simulink model "Steuerung_Modell"  (R2021a)
settings: Solver=FixedStepAuto  StartTime=0.0  StopTime=inf  FixedStep=0.01  MaxStep=0.01  RelTol=1e-3
libraries: simulink x2
settings Model: EnablePacing=on  PacingRate=1.400000  Creator=nymla  LastModifiedBy=nymla

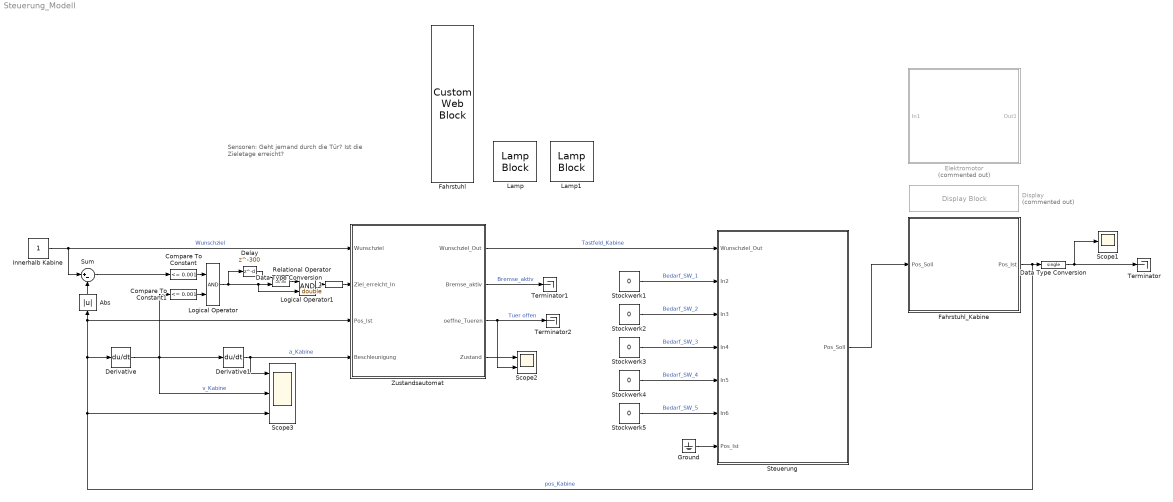
== system Steuerung_Modell ==
  note: Sensoren:
      | Geht jemand durch die Tür?
      | Ist die Zieletage erreicht?
  Abs : Abs
  Compare To Constant : simulink/Logic and Bit Operations/Compare To Constant  relop=<=  const=0.001  OutDataTypeStr=boolean
  Compare To Constant1 : simulink/Logic and Bit Operations/Compare To Constant  relop=<=  const=0.001  OutDataTypeStr=boolean
  Data Type Conversion : DataTypeConversion  OutDataTypeStr=single  RndMeth=Round
  Data Type Conversion1 : DataTypeConversion  OutDataTypeStr=double
  Delay : Delay  DelayLength=300  InitialCondition=1
  Derivative : Derivative
  Derivative1 : Derivative
  Display : DisplayBlock  Commented=on  LabelPosition=Hide  Format=short  Transparency=1
  Elektromotor : Subsystem  Commented=on
  Fahrstuhl : CustomWebBlock  LabelPosition=Hide  ShowInitialText=on  Configuration="{\"components\":[{\"name\":\"LinearScaleComponent\",\"settings\":{\"bounds\":{\"max\":5,\"min\":0,\"tickInterval\":\"auto\"},\"internalTickHeightScaleFactor\":0.5,\"labelColor\":[255,255,200],\"labelFont\":{\"font\":\"Arial\",\"fontSize\":12},\"labelTransparency\":1,\"needleImage\":{\"size\":[21,75],\"src\":\"data:image\\/svg+xml;base64,PHN2ZyB4bWxucz0iaHR0cDovL3d3dy53My5vcmcvMjAwMC9zdmciIHhtbG5zOnhsaW5rPSJodHRwOi8vd3d3LnczLm9yZy8xOTk5L3hsaW5rIiB2aWV3Qm94PSIwIDAgMjEgNzUiPjxkZWZzPjxzdHlsZT4uY2xzLTF7ZmlsbDpub25lO30uY2xzLTJ7aXNvbGF0aW9uOmlzb2xhdGU7fS5jbHMtM3tjbGlwLXBhdGg6dXJsKCNjbGlwLXBhdGgpO30uY2xzLTR7b3BhY2l0eTowLjM7bWl4LWJsZW5kLW1vZGU6bXVsdGlwbHk7fS5jbHMtNXtmaWxsOiNlYjI2Mjk7fTwvc3R5bGU+PGNsaXBQYXRoIGlkPSJjbGlwLXBhdGgiIHRyYW5zZm9y ...(+1928 chars)\",\"srcOrientation\":\"horizontal\"},\"needleOffset\":[-0.01094391244870041,0],\"needleSize\":{\"height\":0.11960078534031414,\"width\":0.7589285714285714},\"position\":[0.015887605042016806,0.06986607142857143,0.8,0.9641544117647058],\"scaleColors\":[],\"scaleColorsSize\":0.2,\"showLabels\":1,\"showMinorTicks\":0,\"showSpanLine\":1,\"showTicks\":1,\"tickColor\":[252,252,197],\"tickTransparency\":1,\"valueBarColor\":[23,89,176],\"valueBarOffset\":0,\"valueBarSize\":0.23,\"valueBarTransparency\":1}},{\"name\":\"BackgroundImageComponent\",\"settings\":{\"image\":{\"size\":[101,380],\"src\":\"data:image\\/svg+xml;base64,PHN2ZyB4bWxucz0iaHR0cDovL3d3dy53My5vcmcvMjAwMC9zdmciIHZpZXdCb3g9IjAgMCAxMDEgMzgwIj48ZGVmcz48c3R5bGU+LmNscy0xe2ZpbGw6IzAwMmI0Mjt9LmNscy0ye2ZpbGw6IzQyNzA4Mjt9LmNscy0ze2ZpbGw6IzdjYTBiMjt9PC9zdHlsZT48L2RlZnM+PHRpdGxlPnZlcnRpY2FsX2dhdWdlX2JhY2tncm91bmRfMTwvdGl0bGU+PGcgaWQ9IkxheWVyXzIiIGRhdGEtbmFtZT0iTGF5ZXIgMiI+PGcgaWQ9IkxheWVyXzEtMiIgZGF0YS1uYW1lPSJMYXllciAxIj48cmVjdCBjbGFzcz0iY2xzLTEiIHg9IjExIiB5PSIxMSIgd2lkdGg9Ijc5IiBoZWlnaHQ9IjM1OCIvPjxwYXRoIGNsYXNzPSJjbHMtMiIgZD0iTTkzLDhIOFYzNzJIOTNaTTExLDM2OVYxMUg5MFYzNjlaIi8+PHBhdGggY2xhc3M9ImNscy0zIiBkPSJNMTAxLDBIMFYzODBIMTAxWk04LDM3MlY4SDkzVjM3MloiLz48L2c+PC9nPjwvc3ZnPg==\",\"srcOrientation\":\"vertical\"},\"position\":[0,0,1,1],\"scaleMode\":\"0\"}},{\"name\":\"ForegroundImageComponent\",\"settings\":{\"image\":{\"size\":[0,0],\"src\":\"default\",\"srcOrientation\":[]},\"isForeground\":1,\"position\":[0,0,1,1],\"scaleMode\":\"0\"}}],\"settings\":{\"BindingType\":\"signal\",\"backgroundColor\":[0,0,0,\"1\"],\"backgroundOffset\":0,\"backgroundOpacity\":1,\"fixedAspectRatio\":\"on\",\"orientation\":\"vertical\",\"showBackgroundColor\":false,\"value\":0},\"type\":\"LinearGauge\"}"
  Fahrstuhl_Kabine : Subsystem
  Ground : Ground
  Innerhalb Kabine : Constant
  Lamp : LampBlock
  Lamp1 : LampBlock
  Logical Operator : Logic  AllPortsSameDT=off  OutDataTypeStr=boolean
  Logical Operator1 : Logic  AllPortsSameDT=off  OutDataTypeStr=boolean
  Relational Operator : RelationalOperator  Operator===  OutDataTypeStr=boolean  RndMeth=Simplest
  Scope1 : Scope
  Scope2 : Scope  NumInputPorts=2
  Scope3 : Scope  NumInputPorts=3
  Steuerung : Subsystem
  Stockwerk{1..5} (5 alike) : Constant  Value=0  OutDataTypeStr=boolean
  Sum : Sum  Inputs=|+-
  Terminator : Terminator
  Terminator1 : Terminator
  Terminator2 : Terminator
  Zustandsautomat : Stateflow chart  TreatAsAtomicUnit=on
      settings: PortSchema="{\"entries\":[{\"content\":{\"sides\":[{\"content\":{\"connectorIds\":[\"In4\",\"In2\",\"In1\",\"In3\"]},\"type\":\"ConnectorPlacement.EquallySpacedRectSide\",\"uuid\":\"96fb556c-ec10-4e34-b155-53f407309d43\"},{\"content\":{\"connectorIds\":[\"Out1\",\"Out2\",\"Out3\",\"Out4\"],\"side\":\"RIGHT\"},\"type\":\"ConnectorPlacement.EquallySpacedRectSide\",\"uuid\":\"cdc6e48a-25d0-4f93-b91a-6f418b4d8265\"},{\"content\":{\"connectorIds\":[],\"side\":\"TOP\"},\"type\":\"ConnectorPlacement.EquallySpacedRectSide\",\"uuid\":\"e64fd8ee-8f58-4024-8019-4a3f9d2aa8c2\"}]},\"type\":\"ConnectorPlacement.EquallySpacedConnector\",\"uuid\":\"deee374e-55c7-4498-8a28-192f5d0177c0\"}],\"packageUris\":[\"http://schema.mathworks.com/mf0/Connector/R2020b\"],\"version\":\"1.0\"}"
  wires:
  Zustandsautomat/1(Wunschziel_Out) -> Steuerung/1(Wunschziel_Out)  "Tastfeld_Kabine"
  Steuerung/1(Pos_Soll) -> Fahrstuhl_Kabine/1(Pos_Soll)
  Fahrstuhl_Kabine/1(Pos_Ist) -> Derivative/1, Zustandsautomat/1(Pos_Ist), Abs/1, Scope3/3, Data Type Conversion/1  "pos_Kabine"
  Data Type Conversion/1 -> Scope1/1, Terminator/1
  Stockwerk2/1 -> Steuerung/3(In3)  "Bedarf_SW_2"
  Stockwerk3/1 -> Steuerung/4(In4)  "Bedarf_SW_3"
  Stockwerk4/1 -> Steuerung/5(In5)  "Bedarf_SW_4"
  Stockwerk5/1 -> Steuerung/6(In6)  "Bedarf_SW_5"
  Stockwerk1/1 -> Steuerung/2(In2)  "Bedarf_SW_1"
  Innerhalb Kabine/1 -> Zustandsautomat/4(Wunschziel), Sum/1  "Wunschziel"
  Derivative/1 -> Scope3/2, Derivative1/1, Compare To Constant1/1  "v_Kabine"
  Derivative1/1 -> Zustandsautomat/3(Beschleunigung), Scope3/1  "a_Kabine"
  Zustandsautomat/4(Zustand) -> Scope2/1
  Sum/1 -> Compare To Constant/1
  Compare To Constant/1 -> Logical Operator/1
  Compare To Constant1/1 -> Logical Operator/2
  Logical Operator/1 -> Relational Operator/2, Logical Operator1/2, Delay/1
  Abs/1 -> Sum/2
  Zustandsautomat/2(Bremse_aktiv) -> Terminator1/1  "Bremse_aktiv"
  Zustandsautomat/3(oeffne_Tueren) -> Terminator2/1, Scope2/2  "Tuer offen"
  Delay/1 -> Relational Operator/1
  Relational Operator/1 -> Logical Operator1/1
  Data Type Conversion1/1 -> Zustandsautomat/2(Ziel_erreicht_In)
  Logical Operator1/1 -> Data Type Conversion1/1
  Ground/1 -> Steuerung/7(Pos_Ist)

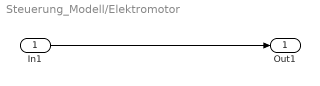
== system Steuerung_Modell/Elektromotor ==
  In1 : Inport
  Out1 : Outport
  wires:
  In1/1 -> Out1/1

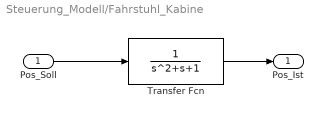
== system Steuerung_Modell/Fahrstuhl_Kabine ==
  Pos_Soll : Inport
  Transfer Fcn : TransferFcn  Denominator=[1 1 1]
  Pos_Ist : Outport
  wires:
  Pos_Soll/1 -> Transfer Fcn/1
  Transfer Fcn/1 -> Pos_Ist/1

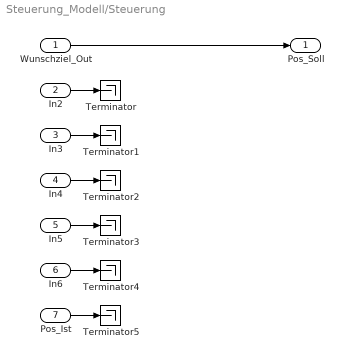
== system Steuerung_Modell/Steuerung ==
  Wunschziel_Out : Inport
  In2 : Inport  Port=2
  In3 : Inport  Port=3
  In4 : Inport  Port=4
  In5 : Inport  Port=5
  In6 : Inport  Port=6
  Pos_Ist : Inport  Port=7
  Terminator{,1..5} (6 alike) : Terminator
  Pos_Soll : Outport
  wires:
  Wunschziel_Out/1 -> Pos_Soll/1
  In2/1 -> Terminator/1
  In3/1 -> Terminator1/1
  In5/1 -> Terminator3/1
  In4/1 -> Terminator2/1
  Pos_Ist/1 -> Terminator5/1
  In6/1 -> Terminator4/1

== stateflow chart Steuerung_Modell/Zustandsautomat ==
  state Fahrstuhl_wartet
    entry:
    Bremse_aktiv = 1;
    Wunschziel_Out = Wunschziel;
    Zustand = 1;
    Ziel_erreicht = Ziel_erreicht_In;
    during:
    Wunschziel_Out = Wunschziel;
  state Tuer_schliessen
    entry:
    oeffne_Tueren=0;
    Zustand = 8;
  state Kabine_beschleunigt
    entry:
    Ziel_erreicht = 0;
    Zustand = 2;
    Bremse_aktiv = 0;
  state Kabine_am_Ziel
    entry:
    Bremse_aktiv = 1;
    Zustand = 6;
    % Hier könnten wir die Bremse
    % entweder aktivieren oder das
    % Signal zum Bremsen geben
  state Tuer_oeffnet
    entry:
    oeffne_Tueren=1;
    Zustand = 7;
  state Kabine_in_Fahrt
    entry:
    Zustand = 3;
  state Schleichfahrt
    entry:
    Zustand = 5;
    Ziel_erreicht = Ziel_erreicht_In;
  state Kabine_bremst_ab
    entry:
    Zustand = 4;
  (default) -> Fahrstuhl_wartet
  Fahrstuhl_wartet -> (junction 81) [order 3]
  Fahrstuhl_wartet -> (junction 89) [order 4]
  Fahrstuhl_wartet -> Fahrstuhl_wartet [order 2] : [Ziel_erreicht ~= Ziel_erreicht_In]
  Fahrstuhl_wartet -> Kabine_beschleunigt [order 1] : [Ziel_erreicht==0]
  Tuer_schliessen -> Fahrstuhl_wartet : after(2,sec)
  Tuer_oeffnet -> Tuer_schliessen : after(15,sec)
  Kabine_beschleunigt -> Kabine_beschleunigt [order 1] : [Beschleunigung>0.1]
  Kabine_beschleunigt -> Kabine_in_Fahrt [order 2] : [Beschleunigung<0.1]
  Kabine_am_Ziel -> Tuer_oeffnet : after(2,sec)
  Schleichfahrt -> Kabine_am_Ziel [order 1] : [Ziel_erreicht==1]
  Kabine_in_Fahrt -> Kabine_in_Fahrt [order 1] : [Beschleunigung<0.1 && Beschleunigung>0]
  Schleichfahrt -> Schleichfahrt [order 2] : [Beschleunigung>-0.1 && Beschleunigung<0.1]
  Kabine_in_Fahrt -> Kabine_bremst_ab [order 2] : [Beschleunigung<-0.001]
  Kabine_bremst_ab -> Kabine_bremst_ab [order 1] : [Beschleunigung<-0.1]
  Kabine_bremst_ab -> Schleichfahrt [order 2] : [Beschleunigung>-0.1 && Beschleunigung<0.1]
  data: Wunschziel_Out output; Pos_Ist input; Ziel_erreicht_In input double; Beschleunigung input; Ziel_erreicht local; Bremse_aktiv output; oeffne_Tueren output; Wunschziel input; Zustand output
